simulink library "Get_System_State"  (R2022b)
settings: Solver=VariableStepAuto  StartTime=0.0  StopTime=10.0  RelTol=1e-3
undefined symbols (not defined in the file): Config
libraries: WBToolboxLibrary x2
settings Model: Creator=fdinatale  LastModifiedBy=fdinatale

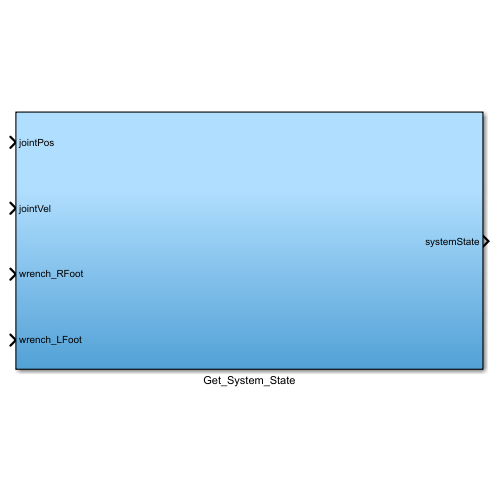
[thumbnail: Simulink's stored preview of the top-level diagram]
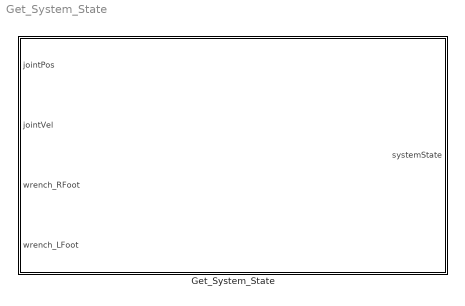
== system Get_System_State ==
  Get_System_State : Subsystem

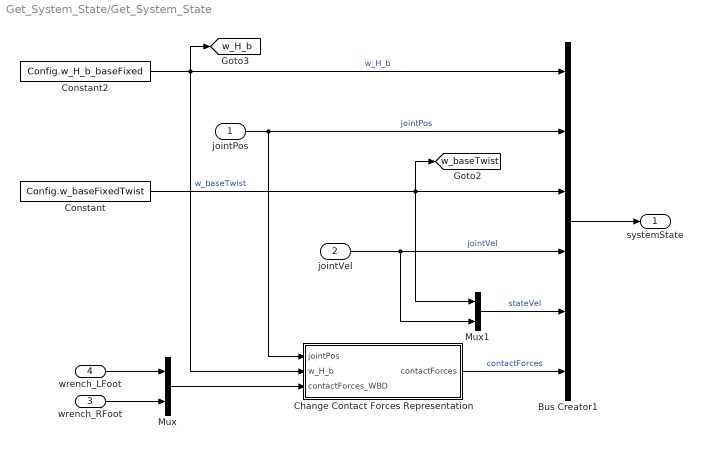
== system Get_System_State/Get_System_State ==
  jointPos : Inport
  jointVel : Inport  Port=2
  wrench_RFoot : Inport  Port=3
  wrench_LFoot : Inport  Port=4
  Bus Creator1 : BusCreator  Inputs=6
  Change Contact Forces Representation : Subsystem
  Constant : Constant  Value=Config.w_baseFixedTwist
  Constant2 : Constant  Value=Config.w_H_b_baseFixed
  Mux : Mux  Inputs=2
  Mux1 : Mux  Inputs=2
  systemState : Outport  VectorParamsAs1DForOutWhenUnconnected=off
  tag scope: w_H_b=global, w_baseTwist=global
  wires:
  Constant2/1 -> Bus Creator1/1, [w_H_b], Change Contact Forces Representation/2(w_H_b)  "w_H_b"
  Bus Creator1/1 -> systemState/1
  Mux/1 -> Change Contact Forces Representation/3(contactForces_WBD)
  Constant/1 -> [w_baseTwist], Mux1/1, Bus Creator1/3  "w_baseTwist"
  jointPos/1 -> Bus Creator1/2, Change Contact Forces Representation/1(jointPos)  "jointPos"
  wrench_LFoot/1 -> Mux/1
  jointVel/1 -> Mux1/2, Bus Creator1/4  "jointVel"
  wrench_RFoot/1 -> Mux/2
  Change Contact Forces Representation/1(contactForces) -> Bus Creator1/6  "contactForces"
  Mux1/1 -> Bus Creator1/5  "stateVel"

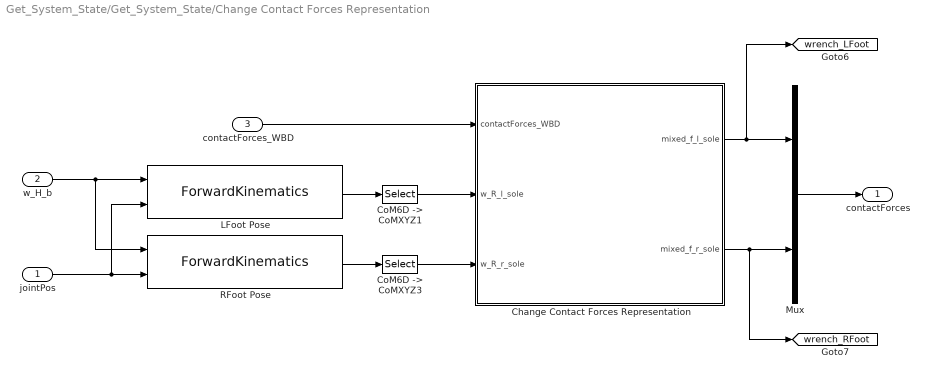
== system Get_System_State/Get_System_State/Change Contact Forces Representation ==
  jointPos : Inport
  w_H_b : Inport  Port=2
  contactForces_WBD : Inport  Port=3
  Change Contact Forces Representation : MATLAB Function  TreatAsAtomicUnit=on
  "CoM6D -> CoMXYZ1" : Selector  NumberOfDimensions=2  InputPortWidth=7  IndexOptions=Index vector (dialog),Index vector (dialog)  Indices=[1 2 3],[1 2 3]  OutputSizes=1,1
  "CoM6D -> CoMXYZ3" : Selector  NumberOfDimensions=2  InputPortWidth=7  IndexOptions=Index vector (dialog),Index vector (dialog)  Indices=[1 2 3],[1 2 3]  OutputSizes=1,1
  LFoot Pose : WBToolboxLibrary/Model/Kinematics/ForwardKinematics  frameName=Frames.LFOOT_FRAME
      settings: SourceProductName=WholeBodyToolbox
  Mux : Mux  Inputs=2
  RFoot Pose : WBToolboxLibrary/Model/Kinematics/ForwardKinematics  frameName=Frames.RFOOT_FRAME
      settings: SourceProductName=WholeBodyToolbox
  contactForces : Outport  VectorParamsAs1DForOutWhenUnconnected=off
  tag scope: wrench_LFoot=global, wrench_RFoot=global
  wires:
  contactForces_WBD/1 -> Change Contact Forces Representation/1(contactForces_WBD)
  RFoot Pose/1 -> "CoM6D -> CoMXYZ3"/1
  "CoM6D -> CoMXYZ3"/1 -> Change Contact Forces Representation/3(w_R_r_sole)
  LFoot Pose/1 -> "CoM6D -> CoMXYZ1"/1
  "CoM6D -> CoMXYZ1"/1 -> Change Contact Forces Representation/2(w_R_l_sole)
  w_H_b/1 -> LFoot Pose/1, RFoot Pose/1
  jointPos/1 -> LFoot Pose/2, RFoot Pose/2
  Change Contact Forces Representation/1(mixed_f_l_sole) -> [wrench_LFoot], Mux/1
  Change Contact Forces Representation/2(mixed_f_r_sole) -> [wrench_RFoot], Mux/2
  Mux/1 -> contactForces/1

== matlab function Get_System_State/Change Contact Forces Representation/Change Contact Forces Representation ==
  data: contactForces_WBD input; mixed_f_l_sole output; w_R_l_sole input; w_R_r_sole input; mixed_f_r_sole output
function [mixed_f_l_sole,mixed_f_r_sole] = fromBodyFrameToMixed_contactForcesFCN(contactForces_WBD,w_R_l_sole,w_R_r_sole)

    [mixed_f_l_sole,mixed_f_r_sole] = iRonCubLib.fromBodyFrameToMixed_contactForces(contactForces_WBD,w_R_l_sole,w_R_r_sole);
end
